simulink model "SPPMSM_DynoLoadTorque"  (R2022b)
settings: Solver=FixedStepDiscrete  StartTime=0.0  StopTime=SimTime  FixedStep=Ts_Model  RelTol=1e-3
libraries: FMIKit_blocks x4
settings Model: Creator=BEDNASA  LastModifiedBy=HENRIE2
settings SolverCC: AlgebraicLoopSolver=TrustRegion
settings DebuggingCC: UnconnectedInputMsg=warning  UnconnectedOutputMsg=warning  UnconnectedLineMsg=warning  SFMachineParentedDataDiag=warning
settings ModelReferenceCC: EnableRefExpFcnMdlSchedulingChecks=on
settings SFSimCC: SimUserSources="\"C:\\Data\\Projects\\MBD_SPM_SimArch\\tools\\FMIKit\\FMIKit-Simulink-2.9\\src\\FMU.cpp\" \"C:\\Data\\Projects\\MBD_SPM_SimArch\\tools\\FMIKit\\FMIKit-Simulink-2.9\\src\\FMU1.cpp\" \"C:\\Data\\Projects\\MBD_SPM_SimArch\\tools\\FMIKit\\FMIKit-Simulink-2.9\\src\\FMU2.cpp\""  SimUserIncludeDirs="\"C:\\Data\\Projects\\MBD_SPM_SimArch\\tools\\FMIKit\\FMIKit-Simulink-2.9\\include\""
settings RTWCC: CustomInclude="\"C:\\Users\\BEDNASA\\Desktop\\SPPMSM\\SPPMSM\\SinglePhaseSimArch_alpha\\tools\\FMIKit-Simulink-2.8\\include\" \"C:\\Users\\BEDNASA\\Desktop\\VA_PSCSimulationArchitecture (2)\\VA_PSCSimulationArchitecture\\tools\\FMIKit-Simulink-2.7\\include\" \"C:\\Users\\BEDNASA\\Desktop\\SPPMSM\\SPPMSM\\MBD_SPM_SimArch\\tools\\include\" \"C:\\Users\\BEDNASA\\Desktop\\SPPMSM\\SPPMSM\\MBD_SPM_SimArch\\tools\\FMIKit\\FMIKit-Simulink-2.9\\include\" \"C:\\Data\\MBD_SPM_SimArch\\tools\\FMIKit\\FMIKit-Simulink-2.9\\include\" \"C:\\Users\\BEDNASA\\Desktop\\Projects\\MBD_SPM_SimArch_v02beta\\MBD_SPM_SimArch\\tools\\FMIKit\\FMIKit-Simulink-2.9\\include\" \"C:\\Data\\Szymon_Projects\\MBD_SPM_SimArch\\tools\\FMIKit\\FMIKit-Simulink-2.9\\include\" \"C:\\Data\\MBD_SPM_SimArch_TEST3\\tools\\FMIKit\\FMIKit-Simulink-2.9\\include\" \"C:\\Data\\Projects\\MBD_SPM_SimArch\\tools\\FMIKit\\FMIKit-Simulink-2.9\\include\""  CustomSource="\"C:\\Users\\BEDNASA\\Desktop\\SPPMSM\\SPPMSM\\SinglePhaseSimArch_alpha\\tools\\FMIKit-Simulink-2.8\\src\\FMU.cpp\" \"C:\\Users\\BEDNASA\\Desktop\\SPPMSM\\SPPMSM\\SinglePhaseSimArch_alpha\\tools\\FMIKit-Simulink-2.8\\src\\FMU1.cpp\" \"C:\\Users\\BEDNASA\\Desktop\\SPPMSM\\SPPMSM\\SinglePhaseSimArch_alpha\\tools\\FMIKit-Simulink-2.8\\src\\FMU2.cpp\" \"C:\\Users\\BEDNASA\\Desktop\\VA_PSCSimulationArchitecture (2)\\VA_PSCSimulationArchitecture\\tools\\FMIKit-Simulink-2.7\\src\\FMU.cpp\" \"C:\\Users\\BEDNASA\\Desktop\\VA_PSCSimulationArchitecture (2)\\VA_PSCSimulationArchitecture\\tools\\FMIKit-Simulink-2.7\\src\\FMU1.cpp\" \"C:\\Users\\BEDNASA\\Desktop\\VA_PSCSimulationArchitecture (2)\\VA_PSCSimulationArchitecture\\tools\\FMIKit-Simulink-2.7\\src\\FMU2.cpp\" \"C:\\Users\\BEDNASA\\Desktop\\SPPMSM\\SPPMSM\\MBD_SPM_SimArch\\tools\\src\\FMU.cpp\" \"C:\\Users\\BEDNASA\\Desktop\\SPPMSM\\SPPMSM\\MBD_SPM_SimArch\\tools\\src\\FMU1.cpp\" \"C:\\Users\\BEDNASA\\Desktop\\SPPMSM\\SPPMSM\\MBD_SPM_SimArch\\tools\\src\\FMU2.cpp\" \"C:\\Users\\BEDNASA\\Desktop\\SPPMSM\\SPPMSM\\MBD_SPM_SimArch\\tools\\FMIKit\\FMIKit-Simulink-2.9\\src\\FMU.cpp\" \"C:\\Users\\BEDNASA\\Desktop\\SPPMSM\\SPPMSM\\MBD_SPM_SimArch\\tools\\FMIKit\\FMIKit-Simulink-2.9\\src\\FMU1.cpp\" \"C:\\Users\\BEDNASA\\Desktop\\SPPMSM\\SPPMSM\\MBD_SPM_SimArch\\tools\\FMIKit\\FMIKit-Simulink-2.9\\src\\FMU2.cpp\" \"C:\\Data\\MBD_SPM_SimArch\\tools\\FMIKit\\FMIKit-Simulink-2.9\\src\\FMU.cpp\" \"C:\\Data\\MBD_SPM_SimArch\\tools\\FMIKit\\FMIKit-Simulink-2.9\\src\\FMU1.cpp\" \"C:\\Data\\MBD_SPM_SimArch\\tools\\FMIKit\\FMIKit-Simulink-2.9\\src\\FMU2.cpp\" \"C:\\Users\\BEDNASA\\Desktop\\Projects\\MBD_SPM_SimArch_v02beta\\MBD_SPM_SimArch\\tools\\FMIKit\\FMIKit-Simulink-2.9\\src\\FMU.cpp\" \"C:\\Users\\BEDNASA\\Desktop\\Projects\\MBD_SPM_SimArch_v02beta\\MBD_SPM_SimArch\\tools\\FMIKit\\FMIKit-Simulink-2.9\\src\\FMU1.cpp\" \"C:\\Users\\BEDNASA\\Desktop\\Projects\\MBD_SPM_SimArch_v02beta\\MBD_SPM_SimArch\\tools\\FMIKit\\FMIKit-Simulink-2.9\\src\\FMU2.cpp\" \"C:\\Data\\Szymon_Projects\\MBD_SPM_SimArch\\tools\\FMIKit\\FMIKit-Simulink-2.9\\src\\FMU.cpp\" \"C:\\Data\\Szymon_Projects\\MBD_SPM_SimArch\\tools\\FMIKit\\FMIKit-Simulink-2.9\\src\\FMU1.cpp\" \"C:\\Data\\Szymon_Projects\\MBD_SPM_SimArch\\tools\\FMIKit\\FMIKit-Simulink-2.9\\src\\FMU2.cpp\" \"C:\\Data\\MBD_SPM_SimArch_TEST3\\tools\\FMIKit\\FMIKit-Simulink-2.9\\src\\FMU.cpp\" \"C:\\Data\\MBD_SPM_SimArch_TEST3\\tools\\FMIKit\\FMIKit-Simulink-2.9\\src\\FMU1.cpp\" \"C:\\Data\\MBD_SPM_SimArch_TEST3\\tools\\FMIKit\\FMIKit-Simulink-2.9\\src\\FMU2.cpp\" \"C:\\Data\\Projects\\MBD_SPM_SimArch\\tools\\FMIKit\\FMIKit-Simulink-2.9\\src\\FMU.cpp\" \"C:\\Data\\Projects\\MBD_SPM_SimArch\\tools\\FMIKit\\FMIKit-Simulink-2.9\\src\\FMU1.cpp\" \"C:\\Data\\Projects\\MBD_SPM_SimArch\\tools\\FMIKit\\FMIKit-Simulink-2.9\\src\\FMU2.cpp\""  CustomLibrary="\"C:\\Program Files\\Microsoft SDKs\\Windows\\v6.0A\\Lib\\x64\\ShLwApi.Lib\""

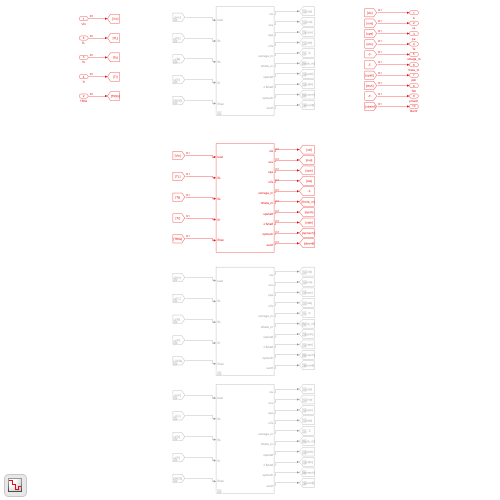
[thumbnail: Simulink's stored preview of the top-level diagram]
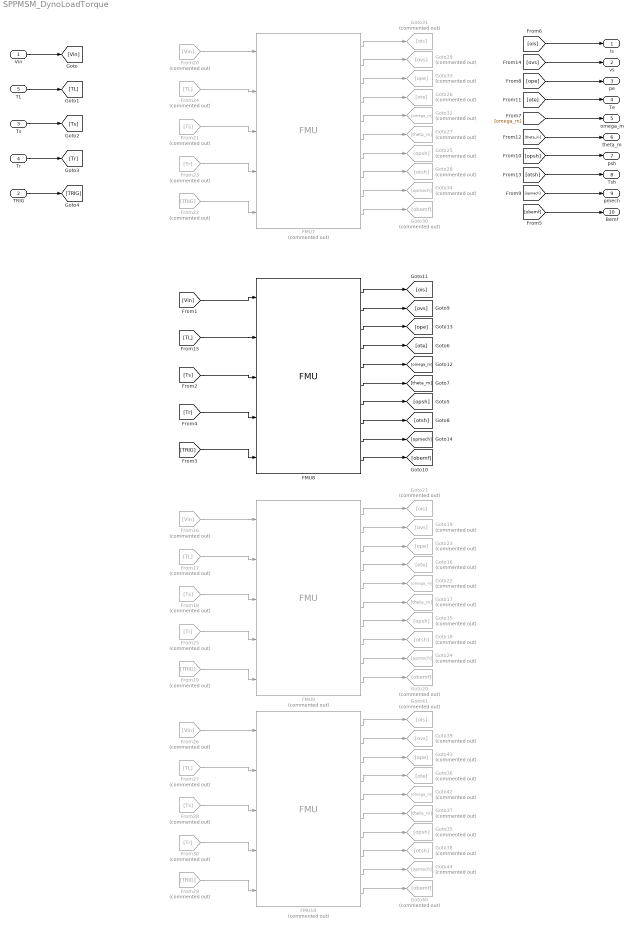
== system SPPMSM_DynoLoadTorque ==
  Vin : Inport
  TRIG : Inport  Port=2
  Ts : Inport  Port=3
  Tr : Inport  Port=4
  TL : Inport  Port=5
  FMU10 : FMIKit_blocks/FMU  Commented=on
      settings: SourceProductName=FMIKit
  FMU7 : FMIKit_blocks/FMU  Commented=on
      settings: SourceProductName=FMIKit
  FMU8 : FMIKit_blocks/FMU
      settings: SourceProductName=FMIKit
  FMU9 : FMIKit_blocks/FMU  Commented=on
      settings: SourceProductName=FMIKit
  From16 : From  Commented=on  GotoTag=Vin
  From17 : From  Commented=on  GotoTag=TL
  From18 : From  Commented=on  GotoTag=Ts
  From19 : From  Commented=on  GotoTag=TRIG
  From20 : From  Commented=on  GotoTag=Vin
  From21 : From  Commented=on  GotoTag=Ts
  From22 : From  Commented=on  GotoTag=TRIG
  From23 : From  Commented=on  GotoTag=Tr
  From24 : From  Commented=on  GotoTag=TL
  From25 : From  Commented=on  GotoTag=Tr
  From26 : From  Commented=on  GotoTag=Vin
  From27 : From  Commented=on  GotoTag=TL
  From28 : From  Commented=on  GotoTag=Ts
  From29 : From  Commented=on  GotoTag=TRIG
  From30 : From  Commented=on  GotoTag=Tr
  Goto15 : Goto  Commented=on  GotoTag=opsh
  Goto16 : Goto  Commented=on  GotoTag=ote
  Goto17 : Goto  Commented=on  GotoTag=theta_m
  Goto18 : Goto  Commented=on  GotoTag=otsh
  Goto19 : Goto  Commented=on  GotoTag=ovs
  Goto20 : Goto  Commented=on  GotoTag=obemf
  Goto21 : Goto  Commented=on  GotoTag=ois
  Goto22 : Goto  Commented=on  GotoTag=omega_m
  Goto23 : Goto  Commented=on  GotoTag=ope
  Goto24 : Goto  Commented=on  GotoTag=opmech
  Goto25 : Goto  Commented=on  GotoTag=opsh
  Goto26 : Goto  Commented=on  GotoTag=ote
  Goto27 : Goto  Commented=on  GotoTag=theta_m
  Goto28 : Goto  Commented=on  GotoTag=otsh
  Goto29 : Goto  Commented=on  GotoTag=ovs
  Goto30 : Goto  Commented=on  GotoTag=obemf
  Goto31 : Goto  Commented=on  GotoTag=ois
  Goto32 : Goto  Commented=on  GotoTag=omega_m
  Goto33 : Goto  Commented=on  GotoTag=ope
  Goto34 : Goto  Commented=on  GotoTag=opmech
  Goto35 : Goto  Commented=on  GotoTag=opsh
  Goto36 : Goto  Commented=on  GotoTag=ote
  Goto37 : Goto  Commented=on  GotoTag=theta_m
  Goto38 : Goto  Commented=on  GotoTag=otsh
  Goto39 : Goto  Commented=on  GotoTag=ovs
  Goto40 : Goto  Commented=on  GotoTag=obemf
  Goto41 : Goto  Commented=on  GotoTag=ois
  Goto42 : Goto  Commented=on  GotoTag=omega_m
  Goto43 : Goto  Commented=on  GotoTag=ope
  Goto44 : Goto  Commented=on  GotoTag=opmech
  is : Outport
  vs : Outport  Port=2
  pe : Outport  Port=3
  Te : Outport  Port=4
  omega_m : Outport  Port=5
  theta_m : Outport  Port=6
  psh : Outport  Port=7
  Tsh : Outport  Port=8
  pmech : Outport  Port=9
  Bemf : Outport  Port=10
  wires:
  Ts/1 -> [Ts]
  TRIG/1 -> [TRIG]
  Vin/1 -> [Vin]
  Tr/1 -> [Tr]
  TL/1 -> [TL]
  [ois] -> is/1
  [ovs] -> vs/1
  [ope] -> pe/1
  [omega_m] -> omega_m/1
  [ote] -> Te/1
  [opmech] -> pmech/1
  [opsh] -> psh/1
  [obemf] -> Bemf/1
  [otsh] -> Tsh/1
  [theta_m] -> theta_m/1
  From23/1 -> FMU7/4
  From24/1 -> FMU7/2
  From21/1 -> FMU7/3
  From20/1 -> FMU7/1
  From22/1 -> FMU7/5
  FMU7/10 -> Goto30/1
  FMU7/9 -> Goto34/1
  FMU7/3 -> Goto33/1
  FMU7/1 -> Goto31/1
  FMU7/5 -> Goto32/1
  FMU7/7 -> Goto25/1
  FMU7/4 -> Goto26/1
  FMU7/6 -> Goto27/1
  FMU7/8 -> Goto28/1
  FMU7/2 -> Goto29/1
  [Vin] -> FMU8/1
  [TL] -> FMU8/2
  [Ts] -> FMU8/3
  [Tr] -> FMU8/4
  [TRIG] -> FMU8/5
  From25/1 -> FMU9/4
  From17/1 -> FMU9/2
  From18/1 -> FMU9/3
  From19/1 -> FMU9/5
  From16/1 -> FMU9/1
  From30/1 -> FMU10/4
  From27/1 -> FMU10/2
  From28/1 -> FMU10/3
  From29/1 -> FMU10/5
  From26/1 -> FMU10/1
  FMU8/7 -> [opsh]
  FMU8/9 -> [opmech]
  FMU8/4 -> [ote]
  FMU8/8 -> [otsh]
  FMU8/5 -> [omega_m]
  FMU8/10 -> [obemf]
  FMU8/2 -> [ovs]
  FMU8/6 -> [theta_m]
  FMU8/3 -> [ope]
  FMU8/1 -> [ois]
  FMU9/7 -> Goto15/1
  FMU9/9 -> Goto24/1
  FMU9/4 -> Goto16/1
  FMU9/8 -> Goto18/1
  FMU9/5 -> Goto22/1
  FMU9/10 -> Goto20/1
  FMU9/2 -> Goto19/1
  FMU9/6 -> Goto17/1
  FMU9/3 -> Goto23/1
  FMU9/1 -> Goto21/1
  FMU10/7 -> Goto35/1
  FMU10/9 -> Goto44/1
  FMU10/4 -> Goto36/1
  FMU10/8 -> Goto38/1
  FMU10/5 -> Goto42/1
  FMU10/10 -> Goto40/1
  FMU10/2 -> Goto39/1
  FMU10/6 -> Goto37/1
  FMU10/3 -> Goto43/1
  FMU10/1 -> Goto41/1
